simulink model "ScanSimilarityRateEstimator_v04"  (R2021a)
settings: Solver=FixedStepAuto  StartTime=0.0  StopTime=inf  RelTol=1e-3
model workspace (MAT data in the model file):
  SL_ROS_VariableLengthArrays_MaxSizes.CommonInfo.ArrayTruncateAction = 'EmitWarning'
  SL_ROS_VariableLengthArrays_MaxSizes.MsgTypeMap = containers.Map
  SL_ROS_VariableLengthArrays_MaxSizes.MsgTypeMap.serialization.keys = {'sensor_msgs/LaserScan'}
  SL_ROS_VariableLengthArrays_MaxSizes.MsgTypeMap.serialization.values{1}(1).PropertyName = 'Intensities'
  SL_ROS_VariableLengthArrays_MaxSizes.MsgTypeMap.serialization.values{1}(1).DataType = 'single'
  SL_ROS_VariableLengthArrays_MaxSizes.MsgTypeMap.serialization.values{1}(1).MaxLength = 1084
  SL_ROS_VariableLengthArrays_MaxSizes.MsgTypeMap.serialization.values{1}(2).PropertyName = 'Ranges'
  SL_ROS_VariableLengthArrays_MaxSizes.MsgTypeMap.serialization.values{1}(2).DataType = 'single'
  SL_ROS_VariableLengthArrays_MaxSizes.MsgTypeMap.serialization.values{1}(2).MaxLength = 1084
  SL_ROS_VariableLengthArrays_MaxSizes.MsgTypeMap.serialization.uniformity = 0
  SL_ROS_VariableLengthArrays_MaxSizes.MsgTypeMap.serialization.keyType = 'char'
  SL_ROS_VariableLengthArrays_MaxSizes.MsgTypeMap.serialization.valueType = 'any'
libraries: robotlib x7
settings Model: Creator=roboticlab01  LastModifiedBy=roboticlab02
settings SolverCC: AlgebraicLoopSolver=TrustRegion
settings OptimizationCC: EnhancedBackFolding=on  PassReuseOutputArgsAs=Individual arguments  MaxStackSize=64  OptimizeBlockOrder=speed  DifferentSizesBufferReuse=on  OptimizationCustomize=off  EfficientTunableParamExpr=on
settings DebuggingCC: ParameterTunabilityLossMsg=error  SFMachineParentedDataDiag=warning
settings HardwareCC: ProdBitPerPointer=32  ProdBitPerSizeT=32  ProdBitPerPtrDiffT=32  ProdLargestAtomicFloat=None  ProdIntDivRoundTo=Undefined  ProdEndianess=Unspecified  ProdWordSize=32  ProdHWDeviceType=Generic->Unspecified (assume 32-bit Generic)
settings SFSimCC: MATLABDynamicMemAlloc=off  CustomCodeUndefinedFunction=UseInterfaceOnly  SimTargetLang=C++
settings RTWCC: SystemTargetFile=ert.tlc  HardwareBoard=Robot Operating System (ROS)  TLCOptions="-aInlineSetEventsForThisBaseRateFcn=TLC_FALSE -aSuppressMultiTaskScheduler=TLC_FALSE  -aRateBasedStepFcn=0"  TemplateMakefile=ert_default_tmf  GenerateReport=on  Toolchain=Catkin  IncludeHyperlinkInReport=on  LaunchReport=on  TargetLang=C++  GenerateTraceInfo=on  GenerateTraceReport=on  GenerateTraceReportSl=on  GenerateTraceReportSf=on  GenerateTraceReportEml=on
settings CodeAppCC: ForceParamTrailComments=on  IgnoreCustomStorageClasses=off  OperatorAnnotations=on  SimulinkDataObjDesc=on  SFDataObjDesc=on  InsertBlockDesc=on
settings ERTTargetCC: SupportVariableSizeSignals=on

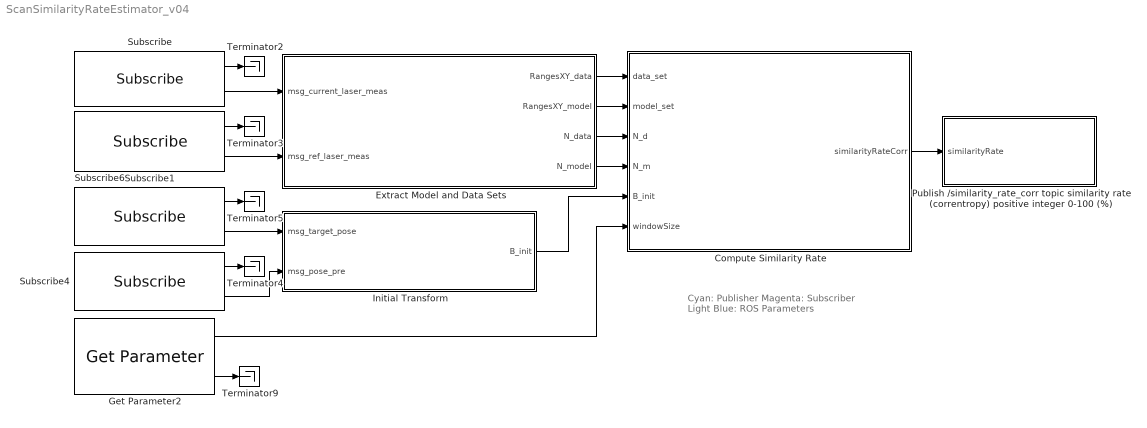
== system ScanSimilarityRateEstimator_v04 ==
  note: Cyan: Publisher
      | Magenta: Subscriber
      | Light Blue: ROS Parameters
  Compute Similarity Rate : Subsystem
  Extract Model and Data Sets : Subsystem
  Get Parameter2 : robotlib/Get Parameter  ParameterSource=Select from ROS network  ParameterName=/windowSize  ParameterType=int32  ParameterMaxArrayLength=16  ParameterInitialValue=10  SampleTime=-1  ShowErrorCodeOutput=on  ModelName=ScanSimilarityRateEstimator_v04  BlockId=ParamGet_ScanSimilarityRateEstimator_v04_541
      settings: SourceProductBaseCode=RR
  Initial Transform : Subsystem
  Publish /similarity_rate_corr topic similarity rate (correntropy) positive integer 0-100 (%) : Subsystem
  Subscribe : robotlib/Subscribe  topicSource=Specify your own  topic=/laser  messageType=sensor_msgs/LaserScan  SampleTime=-1  legacyBusStruct=off  messageQueueLength=1
  Subscribe1 : robotlib/Subscribe  topicSource=Specify your own  topic=/laser_ref  messageType=sensor_msgs/LaserScan  SampleTime=-1  legacyBusStruct=off  messageQueueLength=1
  Subscribe4 : robotlib/Subscribe  topicSource=Specify your own  topic=/current_pose  messageType=geometry_msgs/PoseWithCovarianceStamped  SampleTime=-1  legacyBusStruct=off  messageQueueLength=1
      settings: SourceProductBaseCode=RO
  Subscribe6 : robotlib/Subscribe  topicSource=Select from ROS network  topic=/target_pose  messageType=geometry_msgs/Pose2D  SampleTime=-1  legacyBusStruct=off  messageQueueLength=1
      settings: SourceProductBaseCode=RO
  Terminator{2..5,9} (5 alike) : Terminator
  wires:
  Subscribe/1 -> Terminator2/1
  Subscribe1/1 -> Terminator3/1
  Subscribe4/1 -> Terminator4/1
  Subscribe6/1 -> Terminator5/1
  Compute Similarity Rate/1(similarityRateCorr) -> Publish /similarity_rate_corr topic similarity rate (correntropy) positive integer 0-100 (%)/1(similarityRate)
  Subscribe6/2 -> Initial Transform/1(msg_target_pose)
  Subscribe4/2 -> Initial Transform/2(msg_pose_pre)
  Initial Transform/1(B_init) -> Compute Similarity Rate/5(B_init)
  Subscribe/2 -> Extract Model and Data Sets/1(msg_current_laser_meas)
  Subscribe1/2 -> Extract Model and Data Sets/2(msg_ref_laser_meas)
  Extract Model and Data Sets/1(RangesXY_data) -> Compute Similarity Rate/1(data_set)
  Extract Model and Data Sets/2(RangesXY_model) -> Compute Similarity Rate/2(model_set)
  Extract Model and Data Sets/3(N_data) -> Compute Similarity Rate/3(N_d)
  Extract Model and Data Sets/4(N_model) -> Compute Similarity Rate/4(N_m)
  Get Parameter2/2 -> Terminator9/1
  Get Parameter2/1 -> Compute Similarity Rate/6(windowSize)

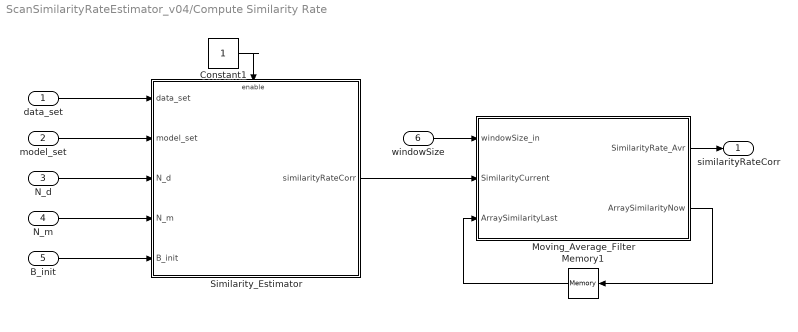
== system ScanSimilarityRateEstimator_v04/Compute Similarity Rate ==
  data_set : Inport
  model_set : Inport  Port=2
  N_d : Inport  Port=3
  N_m : Inport  Port=4
  B_init : Inport  Port=5
  windowSize : Inport  Port=6
  Constant1 : Constant
  Memory1 : Memory  InitialCondition=zeros(50,1)
  Moving_Average_Filter : MATLAB Function  TreatAsAtomicUnit=on
  Similarity_Estimator : Subsystem  TreatAsAtomicUnit=on
  similarityRateCorr : Outport
  wires:
  data_set/1 -> Similarity_Estimator/1(data_set)
  B_init/1 -> Similarity_Estimator/5(B_init)
  model_set/1 -> Similarity_Estimator/2(model_set)
  N_m/1 -> Similarity_Estimator/4(N_m)
  N_d/1 -> Similarity_Estimator/3(N_d)
  Constant1/1 -> Similarity_Estimator/Enable
  Moving_Average_Filter/1(SimilarityRate_Avr) -> similarityRateCorr/1
  Similarity_Estimator/1(similarityRateCorr) -> Moving_Average_Filter/2(SimilarityCurrent)
  Moving_Average_Filter/2(ArraySimilarityNow) -> Memory1/1
  Memory1/1 -> Moving_Average_Filter/3(ArraySimilarityLast)
  windowSize/1 -> Moving_Average_Filter/1(windowSize_in)

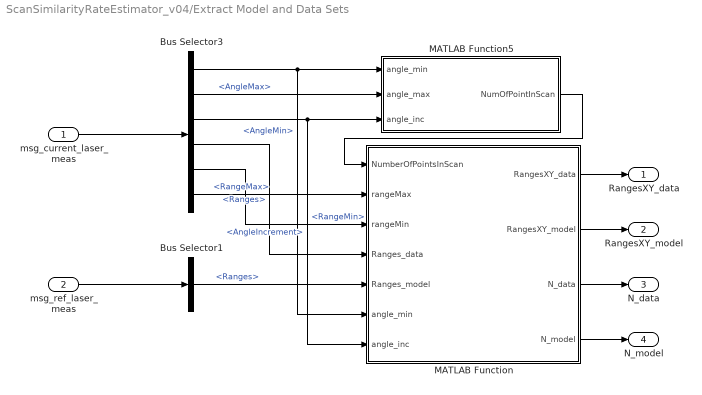
== system ScanSimilarityRateEstimator_v04/Extract Model and Data Sets ==
  msg_current_laser_meas : Inport
  msg_ref_laser_meas : Inport  Port=2
  Bus Selector1 : BusSelector  OutputSignals=Ranges
  Bus Selector3 : BusSelector  OutputSignals=AngleMin,AngleMax,AngleIncrement,Ranges,RangeMin,RangeMax
  MATLAB Function : MATLAB Function  TreatAsAtomicUnit=on
  MATLAB Function5 : MATLAB Function  TreatAsAtomicUnit=on
  RangesXY_data : Outport
  RangesXY_model : Outport  Port=2
  N_data : Outport  Port=3
  N_model : Outport  Port=4
  wires:
  MATLAB Function/1(RangesXY_data) -> RangesXY_data/1
  Bus Selector3/6 -> MATLAB Function/2(rangeMax)  "<RangeMax>"
  MATLAB Function5/1(NumOfPointInScan) -> MATLAB Function/1(NumberOfPointsInScan)
  Bus Selector3/1 -> MATLAB Function/6(angle_min), MATLAB Function5/1(angle_min)  "<AngleMin>"
  msg_current_laser_meas/1 -> Bus Selector3/1
  MATLAB Function/2(RangesXY_model) -> RangesXY_model/1
  MATLAB Function/3(N_data) -> N_data/1
  Bus Selector3/4 -> MATLAB Function/4(Ranges_data)  "<Ranges>"
  msg_ref_laser_meas/1 -> Bus Selector1/1
  MATLAB Function/4(N_model) -> N_model/1
  Bus Selector3/5 -> MATLAB Function/3(rangeMin)  "<RangeMin>"
  Bus Selector3/3 -> MATLAB Function/7(angle_inc), MATLAB Function5/3(angle_inc)  "<AngleIncrement>"
  Bus Selector3/2 -> MATLAB Function5/2(angle_max)  "<AngleMax>"
  Bus Selector1/1 -> MATLAB Function/5(Ranges_model)  "<Ranges>"

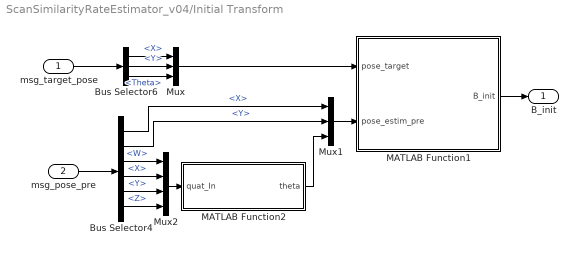
== system ScanSimilarityRateEstimator_v04/Initial Transform ==
  msg_target_pose : Inport
  msg_pose_pre : Inport  Port=2
  Bus Selector4 : BusSelector  OutputSignals=Pose.Pose.Position.X,Pose.Pose.Position.Y,Pose.Pose.Orientation.W,Pose.Pose.Orientation.X,Pose.Pose.Orientation.Y,Pose.Pose.Orientation.Z
  Bus Selector6 : BusSelector  OutputSignals=X,Y,Theta
  MATLAB Function1 : MATLAB Function  TreatAsAtomicUnit=on
  MATLAB Function2 : MATLAB Function  TreatAsAtomicUnit=on
  Mux : Mux  Inputs=3
  Mux1 : Mux  Inputs=3
  Mux2 : Mux
  B_init : Outport
  wires:
  Bus Selector6/2 -> Mux/2  "<Y>"
  Bus Selector4/3 -> Mux2/1  "<W>"
  Bus Selector4/4 -> Mux2/2  "<X>"
  Mux2/1 -> MATLAB Function2/1(quat_In)
  Bus Selector4/2 -> Mux1/2  "<Y>"
  Bus Selector4/6 -> Mux2/4  "<Z>"
  MATLAB Function2/1(theta) -> Mux1/3
  msg_pose_pre/1 -> Bus Selector4/1
  Bus Selector4/1 -> Mux1/1  "<X>"
  Bus Selector4/5 -> Mux2/3  "<Y>"
  MATLAB Function1/1(B_init) -> B_init/1
  Bus Selector6/3 -> Mux/3  "<Theta>"
  msg_target_pose/1 -> Bus Selector6/1
  Bus Selector6/1 -> Mux/1  "<X>"
  Mux/1 -> MATLAB Function1/1(pose_target)
  Mux1/1 -> MATLAB Function1/2(pose_estim_pre)

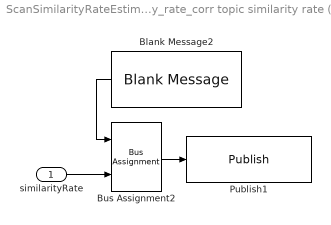
== system ScanSimilarityRateEstimator_v04/Publish //similarity_rate_corr topic similarity rate (correntropy) positive integer 0-100 (%) ==
  similarityRate : Inport
  Blank Message2 : robotlib/Blank Message  messageClass=Message  entityType=std_msgs/Int16  messageType=std_msgs/Int16  SampleTime=inf  legacyBusStruct=off
      settings: SourceProductBaseCode=RO
  Bus Assignment2 : BusAssignment  AssignedSignals=Data
  Publish1 : robotlib/Publish  topicSource=Specify your own  topic=/similarity_rate_corr  messageType=std_msgs/Int16  legacyBusStruct=off  messageQueueLength=1
      settings: SourceProductBaseCode=RO
  wires:
  Bus Assignment2/1 -> Publish1/1
  similarityRate/1 -> Bus Assignment2/2
  Blank Message2/1 -> Bus Assignment2/1

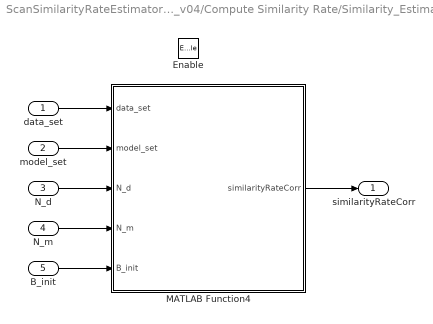
== system ScanSimilarityRateEstimator_v04/Compute Similarity Rate/Similarity_Estimator ==
  data_set : Inport
  model_set : Inport  Port=2
  N_d : Inport  Port=3
  N_m : Inport  Port=4
  B_init : Inport  Port=5
  Enable : EnablePort
  MATLAB Function4 : MATLAB Function  TreatAsAtomicUnit=on
  similarityRateCorr : Outport
  wires:
  data_set/1 -> MATLAB Function4/1(data_set)
  model_set/1 -> MATLAB Function4/2(model_set)
  N_d/1 -> MATLAB Function4/3(N_d)
  N_m/1 -> MATLAB Function4/4(N_m)
  B_init/1 -> MATLAB Function4/5(B_init)
  MATLAB Function4/1(similarityRateCorr) -> similarityRateCorr/1

== matlab function ScanSimilarityRateEstimator_v04/Initial Transform/MATLAB Function1 ==
  data: pose_target input; B_init output [..2000]; pose_estim_pre input
function B_init = Initial_tf(pose_target,pose_estim_pre)

    th_B = wrapTo360(pose_estim_pre(3,1)-pose_target(3,1));
    R_trgt2ref_cf = [cosd(pose_target(3,1)),-sind(pose_target(3,1));sind(pose_target(3,1)),cosd(pose_target(3,1))];
    t_B = R_trgt2ref_cf'*(pose_estim_pre(1:2,1) - pose_target(1:2,1));
    B_init = rotz(th_B);
    B_init(1:2,3) = t_B;

end

== matlab function ScanSimilarityRateEstimator_v04/Extract Model and Data Sets/MATLAB Function ==
  data: NumberOfPointsInScan input size=1 [..2000]; rangeMax input; rangeMin input; Ranges_data input; Ranges_model input; RangesXY_data output double size=[2,2000]; angle_min input; angle_inc input; RangesXY_model output size=[2,2000]; N_data output size=1 [..2000]; N_model output size=1 [..2000]
function [RangesXY_data,RangesXY_model,N_data,N_model] = Model_Data_Extract(NumberOfPointsInScan,rangeMax,rangeMin,Ranges_data,Ranges_model,angle_min,angle_inc)
    
    N_model = 0;
    N_data = 0;

    if ~isnan(NumberOfPointsInScan)
        Ranges_data(Ranges_data < rangeMin | Ranges_data > rangeMax) = NaN;
        Ranges_model(Ranges_model < rangeMin | Ranges_model > rangeMax) = NaN;
        Ranges_Used_data = double(Ranges_data');            
        RangesXY_data = NaN(2,size(Ranges_Used_data,2));
        Ranges_Used_model = double(Ranges_model');          
        RangesXY_model = NaN(2,size(Ranges_Used_model,2));   
    
        for i = 1:1:NumberOfPointsInScan
            if isinf(Ranges_Used_data(1,i))
               Ranges_Used_data(1,i) = NaN;  
            end
            RangesXY_data(:,i) = Ranges_Used_data(1,i)*[cos(angle_min + angle_inc*(i-1));...
                sin(angle_min + angle_inc*(i-1))];
        end
        
        RangesXY_data = sortrows(RangesXY_data')';
        for i = 1:1:NumberOfPointsInScan
            if isnan(RangesXY_data(1,i))
                N_data = i-1;
                break;
            end
        end
        
        for i = 1:1:NumberOfPointsInScan
            if isinf(Ranges_Used_model(1,i))
               Ranges_Used_model(1,i) = NaN;  
            end
            RangesXY_model(:,i) = Ranges_Used_model(1,i)*[cos(angle_min + angle_inc*(i-1));...
                sin(angle_min + angle_inc*(i-1))];
        end
        
        RangesXY_model = sortrows(RangesXY_model')';
        for i = 1:1:NumberOfPointsInScan
            if isnan(RangesXY_model(1,i))
                N_model = i-1;
                break;
            end
        end
        
    else
        RangesXY_data = [];
        RangesXY_model = [];
    end

== matlab function ScanSimilarityRateEstimator_v04/Initial Transform/MATLAB Function2 ==
  data: quat_In input; theta output size=1 [..2000]
function theta = Quat2Euler(quat_In)

    eul = quat2eul(quat_In');
    eul_deg = rad2deg(eul);
    theta = eul_deg(1,1);
end

== matlab function ScanSimilarityRateEstimator_v04/Compute Similarity Rate/Similarity_Estimator/MATLAB Function4 ==
  data: data_set input size=[2,2000]; model_set input size=[2,2000]; N_d input size=1 [..2000]; N_m input size=1 [..2000]; similarityRateCorr output; B_init input
function similarityRateCorr   = FindSimilarityRate(data_set,model_set,N_d,N_m,B_init)
%%%%%%%%%%%%%%%%%%%%%%%%%%%%%%%%%%%%%%%%%%%%%%%%%%%%%%%%%%%%%%%%%%%%%%%%%%%
%%%%%%%%%%%%%%%%%%%%% Similarity Rate Computation %%%%%%%%%%%%%%%%%%%%%%%%%
%%%%%%%%%%%%%%%%%%%%%%%%%%%%%%%%%%%%%%%%%%%%%%%%%%%%%%%%%%%%%%%%%%%%%%%%%%%
% Author  : Abdurrahman YILMAZ
% Date    : 08.11.2021
% Version : v02
% Notes   : The corresponding points of the model and data sets are 
%  determined to estimate overlap ratio between point sets 
% correntropy based overlap estimator design
%%%%%%%%%%%%%%%%%%%%%%%%%%%%%%%%%%%%%%%%%%%%%%%%%%%%%%%%%%%%%%%%%%%%%%%%%%
        
    B_km1 = B_init;
    
    model_in = model_set';
    data_in = data_set';
        
    N_model = N_m;
    N_data = N_d;
    model= model_in(1:N_model,:);
    M1 = model;
    M = [M1,ones(size(M1,1),1)];
    data = data_in(1:N_data,:);
    P1 = data;
    P = [P1,ones(size(P1,1),1)];
            
    Pbar = (B_km1*P')';
    [Idx_d2m,Dist_d2m] = knnsearch(M(:,1:2),Pbar(:,1:2),'k',1);
        
    corr_points = [double(Idx_d2m),Dist_d2m,Pbar,P];
    corr_points = sortrows(corr_points,2);
    
    median_d2m = median(Dist_d2m);
    
    Dist4sigma = median_d2m + (median_d2m - min(Dist_d2m));
        
    indexId = size(corr_points,1);

    for j = size(corr_points,1):-1:1
        if corr_points(j,2) <= Dist4sigma
            indexId = j;
            break;
        end
    end
    
    sigma = std(Dist_d2m(1:indexId,:));
%         
%     % Draw from 0 to 1 overlap changing trajectory of overlap objective
%     % function
%     zeta = 0.1:0.02:1;
%     S_TS = zeros(1,length(zeta));
%     e = zeros(1,length(zeta));
%     for i = 1:1:length(zeta)
%         N = round(N_data*zeta(i));
%         for j = 1:1:N
%             S_TS(i) = S_TS(i) + exp(-(norm(corr_points(j,2))^2/(2*sigma^2)));
%         end
%         e(i) = S_TS(i)/N;
%     end
%     e_dot = gradient(e(:)) ./ gradient(zeta(:));
        
    zeta_alpha = 0.1; % lower bound
    zeta_beta = 0.99; % upper bound
    w = 1/3;
    
    while(1)
        zeta_1 = zeta_alpha + w*(zeta_beta-zeta_alpha);
        zeta_2 = zeta_beta - w*(zeta_beta-zeta_alpha);
        zetaList = [zeta_alpha,zeta_1,zeta_2,zeta_beta];
        S_TS_list = zeros(1,length(zetaList));
        e_list = zeros(1,length(zetaList));
        for i = 1:1:length(zetaList)
            N = round(N_data*zetaList(i));
            for j = 1:1:N
                S_TS_list(i) = S_TS_list(i) + exp(-(norm(corr_points(j,2))^2/(2*sigma^2)));
            end
            e_list(i) = S_TS_list(i)/N;
        end
        e_list_dot = gradient(e_list(:)) ./ gradient(zetaList(:));
        if e_list_dot(1,1) < e_list_dot(2,1) % kappa_alpha < kappa_zeta_1
            zeta_beta = zeta_1;
        elseif e_list_dot(2,1) < e_list_dot(3,1) % kappa_zeta_1 < kappa_zeta_2
                zeta_beta = zeta_2;
        else
            zeta_alpha = zeta_1;
        end

        if abs(zeta_alpha - zeta_beta) <= 0.01
            similarity_rate = (zeta_alpha + zeta_beta)/2;
            break;
        end
    end
    similarityRateCorr = similarity_rate;

== matlab function ScanSimilarityRateEstimator_v04/Extract Model and Data Sets/MATLAB Function5 ==
  data: angle_min input; NumOfPointInScan output size=1 [..2000]; angle_max input; angle_inc input
function NumOfPointInScan   = ScanInfo(angle_min,angle_max,angle_inc)
    NumOfPointInScan = double(round(abs(angle_max - angle_min)/angle_inc)+1);
end

== matlab function ScanSimilarityRateEstimator_v04/Compute Similarity Rate/Moving_Average_Filter ==
  data: windowSize_in input; SimilarityRate_Avr output; SimilarityCurrent input; ArraySimilarityLast input; ArraySimilarityNow output
function [SimilarityRate_Avr,ArraySimilarityNow]  = MovingAverageSimilarityRate(windowSize_in,SimilarityCurrent,ArraySimilarityLast)
%%%%%%%%%%%%%%%%%%%%%%%%%%%%%%%%%%%%%%%%%%%%%%%%%%%%%%%%%%%%%%%%%%%%%%%%%%%
% Calculate average similarity rate (percentage) for selected window size %
%%%%%%%%%%%%%%%%%%%%%%%%%%%%%%%%%%%%%%%%%%%%%%%%%%%%%%%%%%%%%%%%%%%%%%%%%%%
% Author  : Abdurrahman YILMAZ
% Date    : 08.11.2021
% Version : v01
% Notes   : The last ... similarity rate values are stored and average of
% of similarities over last window size is calculated and published as
% similarity rate
%%%%%%%%%%%%%%%%%%%%%%%%%%%%%%%%%%%%%%%%%%%%%%%%%%%%%%%%%%%%%%%%%%%%%%%%%%
    if isempty(windowSize_in) || isnan(windowSize_in) || isinf(windowSize_in) || windowSize_in <= 0 || windowSize_in >= 50
        windowSize = int32(10); % default value
    else
        windowSize = windowSize_in; % taken as ros parameter
    end

    ArrayOverlapListDummy = ArraySimilarityLast;
    
    ArrayOverlapListDummy = [SimilarityCurrent;ArrayOverlapListDummy(1:end-1,:)];
    
    ArraySimilarityNow = ArrayOverlapListDummy;
    SimilarityRate_Avr = int16(round(mean(nonzeros(ArraySimilarityNow(1:windowSize)))*100));% Average similarity for the selected window size
    
end
